simulink model "ForcePositionCBAgent"  (Simulink 7.1)
settings: Solver=ode45  SolverMode=SingleTasking  StartTime=0.0  StopTime=10.0  RelTol=1e-3  AbsTol=1e-6
settings Model: Creator=The MathWorks Inc.  LastModifiedBy=suarezjl  ExtModeTrigMode=oneshot  ExtModeArmWhenConnect=off  ExtModeAutoUpdateStatusClock=off
settings DataIOCC: LimitDataPoints=off  SignalLoggingName=logsOut
settings OptimizationCC: BooleanDataType=off  InlineInvariantSignals=on
settings DebuggingCC: SaveWithParameterizedLinksMsg=none  CheckExecutionContextPreStartOutputMsg=on  CheckExecutionContextRuntimeOutputMsg=on  SignalResolutionControl=TryResolveAllWithWarning  SolverPrmCheckMsg=none  MultiTaskDSMMsg=warning  MultiTaskCondExecSysMsg=none  IntegerOverflowMsg=none  StrictBusMsg=None
settings HardwareCC: TargetUnknown=on
settings ModelReferenceCC: UpdateModelReferenceTargets=IfOutOfDate
settings RTWCC: IncludeERTFirstTime=on
settings GRTTargetCC: TargetFcnLib=ansi_tfl_tmw.mat

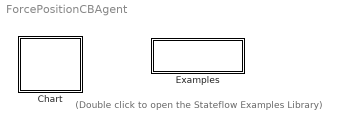
== system ForcePositionCBAgent ==
  note: (Double click to open the
      | Stateflow Examples Library)
  Chart : Stateflow chart
  Examples : Subsystem
      settings: OpenFcn=sf('Private','sf_examples')
      mask Display: disp('Examples')

== system ForcePositionCBAgent/Examples ==

== stateflow chart Chart ==
  state Initialize
    Aquateen\ControlBasisModule\ForcePositionCB\ForcePositionCB.Initialize()
    Aquateen\ControlBasisModule\HP3JCAgent\HP3JC.connect_Initialize()
    Aquateen\ControlBasisModule\HP3JCAgent\HP3JC.servo_ServoOn()
    Aquateen\ControlBasisModule\HP3JCAgent\HP3JC.job_SelectJob()
    Aquateen\ControlBasisModule\HP3JCAgent\HP3JC.job_StartJob()
  state ReadPosition
    Aquateen\ControlBasisModule\HP3JCAgent\HP3JC.read_CurrentPosition()
    Aquateen\ControlBasisModule\ForcePositionCB\ForcePositionCB.ComputeControlBasis()
    Aquateen\ControlBasisModule\HP3JCAgent\HP3JC.move_JointAngles()
  state Stop
    Aquateen\ControlBasisModule\HP3JCAgent\HP3JC.error_ClearError()
    Aquateen\ControlBasisModule\HP3JCAgent\HP3JC.error_ClearAlarm()
    Aquateen\ControlBasisModule\HP3JCAgent\HP3JC.job_SelectJob()
    Aquateen\ControlBasisModule\HP3JCAgent\HP3JC.job_StartJob()
    Aquateen\ControlBasisModule\ForcePositionCB\StateMachine.Wait(500)
    Aquateen\ControlBasisModule\HP3JCAgent\HP3JC.connect_Disconnect()
  (default) -> Initialize : Start
  Initialize -> ReadPosition : Always
  ReadPosition -> ReadPosition [order 1] : Default
  ReadPosition -> Stop [order 2] : Signal="End"
